simulink library "INT_CoTE_ThermDem"  (R2016b)
settings: Solver=VariableStepAuto  StartTime=0.0  StopTime=10.0  RelTol=1e-3
settings Model: Creator=Administrator  LastModifiedBy=Administrator

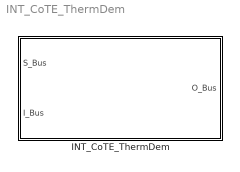
== system INT_CoTE_ThermDem ==
  INT_CoTE_ThermDem : Subsystem

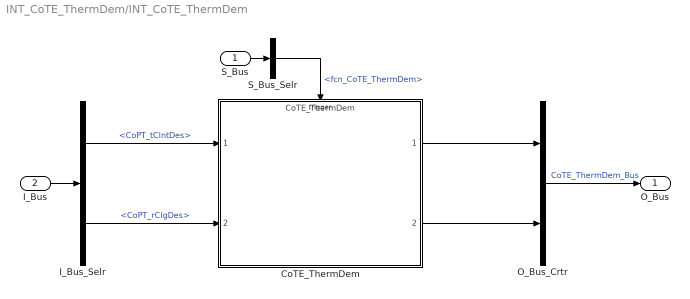
== system INT_CoTE_ThermDem/INT_CoTE_ThermDem ==
  S_Bus : Inport
  I_Bus : Inport  Port=2
  CoTE_ThermDem : ModelReference  ModelNameDialog=CoTE_ThermDem  SimulationMode=Normal  ModelReferenceVersion=1.8  TriggerPortName=function  TriggerPortTriggerType=function-call  TriggerPortStatesWhenEnabling=held
  I_Bus_Selr : BusSelector  OutputSignals=CoPT_tClntDes,CoPT_rClgDes
  O_Bus_Crtr : BusCreator  Inputs=2
  S_Bus_Selr : BusSelector  OutputSignals=fcn_CoTE_ThermDem
  O_Bus : Outport
  wires:
  S_Bus_Selr/1 -> CoTE_ThermDem/Trigger  "<fcn_CoTE_ThermDem>"
  S_Bus/1 -> S_Bus_Selr/1
  I_Bus/1 -> I_Bus_Selr/1
  I_Bus_Selr/1 -> CoTE_ThermDem/1  "<CoPT_tClntDes>"
  I_Bus_Selr/2 -> CoTE_ThermDem/2  "<CoPT_rClgDes>"
  O_Bus_Crtr/1 -> O_Bus/1  "CoTE_ThermDem_Bus"
  CoTE_ThermDem/1 -> O_Bus_Crtr/1
  CoTE_ThermDem/2 -> O_Bus_Crtr/2
